simulink model "data_store_model"  (R2022b)
settings: Solver=VariableStepAuto  StartTime=0.0  StopTime=10.0  RelTol=1e-3
settings Model: Creator=Brigosha_Guest  LastModifiedBy=Brigosha_Guest

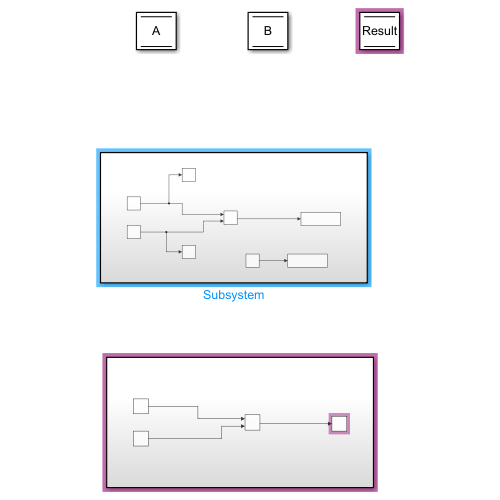
[thumbnail: Simulink's stored preview of the top-level diagram]
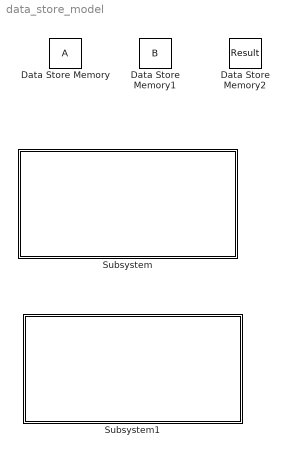
== system data_store_model ==
  Data Store Memory : DataStoreMemory  WriteAfterWriteMsg=warning  ShowAdditionalParam=off
  Data Store Memory1 : DataStoreMemory  DataStoreName=B  WriteAfterWriteMsg=warning  ShowAdditionalParam=off
  Data Store Memory2 : DataStoreMemory  DataStoreName=Result  WriteAfterWriteMsg=warning  ShowAdditionalParam=off
  Subsystem : Subsystem
  Subsystem1 : Subsystem

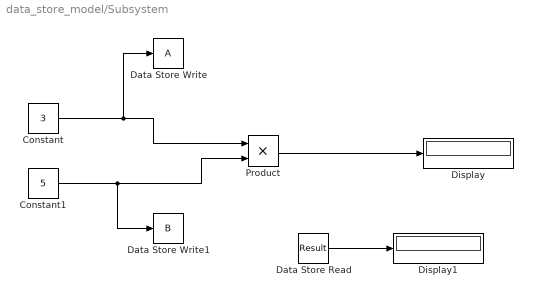
== system data_store_model/Subsystem ==
  Constant : Constant  Value=3
  Constant1 : Constant  Value=5
  Data Store Read : DataStoreRead  DataStoreName=Result  IndexOptions=Index vector (dialog)  Indices=1  OutputSizes=1
  Data Store Write : DataStoreWrite  IndexOptions=Index vector (dialog)  Indices=1  OutputSizes=1
  Data Store Write1 : DataStoreWrite  DataStoreName=B  IndexOptions=Index vector (dialog)  Indices=1  OutputSizes=1
  Display : Display
  Display1 : Display
  Product : Product
  wires:
  Constant1/1 -> Data Store Write1/1, Product/2
  Product/1 -> Display/1
  Constant/1 -> Data Store Write/1, Product/1
  Data Store Read/1 -> Display1/1

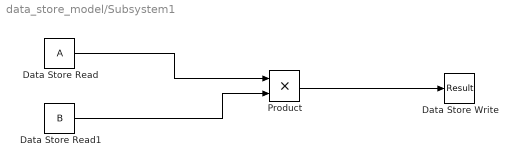
== system data_store_model/Subsystem1 ==
  Data Store Read : DataStoreRead  IndexOptions=Index vector (dialog)  Indices=1  OutputSizes=1
  Data Store Read1 : DataStoreRead  DataStoreName=B  IndexOptions=Index vector (dialog)  Indices=1  OutputSizes=1
  Data Store Write : DataStoreWrite  DataStoreName=Result  IndexOptions=Index vector (dialog)  Indices=1  OutputSizes=1
  Product : Product
  wires:
  Data Store Read/1 -> Product/1
  Product/1 -> Data Store Write/1
  Data Store Read1/1 -> Product/2
